simulink model "Practica1_Debanhi_Rodriguez_DoblePendulo"  (R2022a)
settings: Solver=VariableStepAuto  StartTime=0.0  StopTime=10.0  MaxStep=0.00001  RelTol=1e-3
values from neighbouring files (symbols this model uses):
  g = 9.81    [Parametros_practica_1.m]
  L1 = 0.3    [Parametros_practica_1.m]
  L2 = 0.25    [Parametros_practica_1.m]
  m1 = 0.2    [Parametros_practica_1.m]
  m2 = 0.1    [Parametros_practica_1.m]
settings Model: Creator=patit  LastModifiedBy=patit

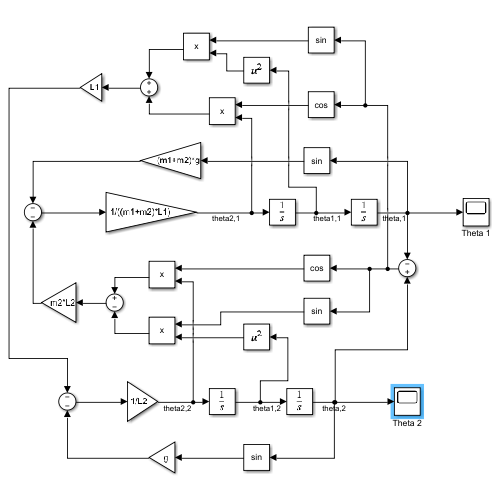
[thumbnail: Simulink's stored preview of the top-level diagram]
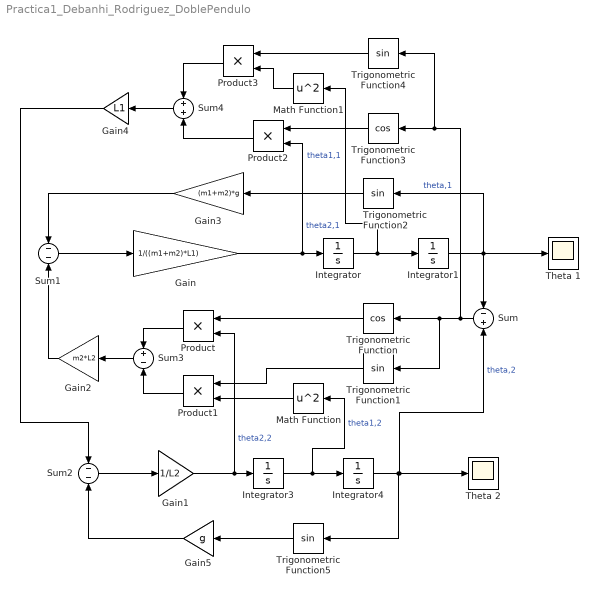
== system Practica1_Debanhi_Rodriguez_DoblePendulo ==
  Gain : Gain  Gain=1/((m1+m2)*L1)
  Gain1 : Gain  Gain=1/L2
  Gain2 : Gain  Gain=m2*L2
  Gain3 : Gain  Gain=(m1+m2)*g
  Gain4 : Gain  Gain=L1
  Gain5 : Gain  Gain=g
  Integrator : Integrator
  Integrator1 : Integrator
  Integrator3 : Integrator
  Integrator4 : Integrator  InitialCondition=(35*pi)/180
  Math Function : Math  Operator=square
  Math Function1 : Math  Operator=square
  Product{,1..3} (4 alike) : Product
  Sum : Sum  Inputs=-+
  Sum1 : Sum  Inputs=--
  Sum2 : Sum  Inputs=--
  Sum3 : Sum  Inputs=+-
  Sum4 : Sum
  Theta 1 : Scope
  Theta 2 : Scope
  Trigonometric Function : Trigonometry  Operator=cos
  Trigonometric Function{1..2,4..5} (4 alike) : Trigonometry
  Trigonometric Function3 : Trigonometry  Operator=cos
  wires:
  Gain/1 -> Product2/2, Integrator/1  "theta2,1"
  Integrator/1 -> Math Function1/1, Integrator1/1  "theta1,1"
  Integrator1/1 -> Theta 1/1, Trigonometric Function2/1, Sum/1  "theta,1"
  Sum1/1 -> Gain/1
  Integrator4/1 -> Trigonometric Function5/1, Theta 2/1, Sum/2  "theta,2"
  Gain1/1 -> Product/2, Integrator3/1  "theta2,2"
  Integrator3/1 -> Math Function/1, Integrator4/1  "theta1,2"
  Sum2/1 -> Gain1/1
  Sum/1 -> Trigonometric Function4/1, Trigonometric Function3/1, Trigonometric Function1/1, Trigonometric Function/1
  Trigonometric Function/1 -> Product/1
  Trigonometric Function1/1 -> Product1/1
  Math Function/1 -> Product1/2
  Product/1 -> Sum3/1
  Product1/1 -> Sum3/2
  Sum3/1 -> Gain2/1
  Gain2/1 -> Sum1/2
  Trigonometric Function2/1 -> Gain3/1
  Gain3/1 -> Sum1/1
  Trigonometric Function3/1 -> Product2/1
  Trigonometric Function4/1 -> Product3/1
  Math Function1/1 -> Product3/2
  Product2/1 -> Sum4/2
  Product3/1 -> Sum4/1
  Sum4/1 -> Gain4/1
  Gain4/1 -> Sum2/1
  Trigonometric Function5/1 -> Gain5/1
  Gain5/1 -> Sum2/2
